simulink model "robot"  (R2021a)
settings: Solver=FixedStepAuto  StartTime=0.0  StopTime=tf  FixedStep=ts  RelTol=ts
PreLoadFcn:
  | robot_data;
InitFcn:
  | robot_data;
values from neighbouring files (symbols this model uses):
  c11 = coefficients_hexic(Theta(1,1), Theta(2,1), Theta(3,1), t1, tf)    [robot_data.m]
  c12 = NaN(size(c11))    [robot_data.m]
  c21 = coefficients_hexic(Theta(1,2), Theta(2,2), Theta(3,2), t1, tf)    [robot_data.m]
  c22 = NaN(size(c21))    [robot_data.m]
  obs = [0.2, 0.1]    [robot_data.m]
  offset = 0.183    [robot_data.m]
  r1 = 0.21    [robot_data.m]
  r2 = 0.2452    [robot_data.m]
  t1 = 4    [robot_data.m]    (also in trajectory_planning.m = 2)
settings Model: EnablePacing=on  Creator=matti  LastModifiedBy=matti

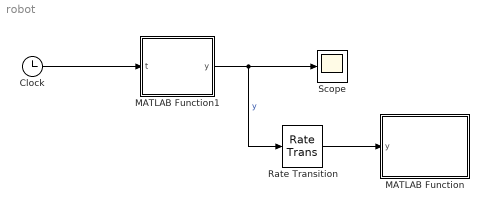
== system robot ==
  Clock : Clock
  MATLAB Function : MATLAB Function  TreatAsAtomicUnit=on
  MATLAB Function1 : MATLAB Function  TreatAsAtomicUnit=on
  Rate Transition : RateTransition  OutPortSampleTime=ts
  Scope : Scope
  wires:
  Rate Transition/1 -> MATLAB Function/1(y)
  Clock/1 -> MATLAB Function1/1(t)
  MATLAB Function1/1(y) -> Rate Transition/1, Scope/1  "y"

== matlab function robot/MATLAB Function ==
  data: y input; r1 parameter; r2 parameter; obs parameter; offset parameter
%% Animation function
function robot_display(y, r1, r2, obs, offset)
% Animation of the robot with the lower and upper arm as well as 
% the shoulder, elbow and hand and the obstacle
% Input     Type        Description
% y         2x1 double  simulation output
% Parameter Type        Description
% r1        1x1 double  upper arm length [m]
% r2        1x1 double  lower arm length [m]
% obs       2x1 double  x-position and height of the obstacle
% offset    1x1 double  y offset of first joint
coder.extrinsic('patch');
persistent upperarm;
persistent lowerarm;
persistent foot;
persistent shoulder;
persistent elbow;
persistent hand;
persistent obstacle;
%% Parameters
width = 0.02;      % width of both arms [m]
w2 = width/2;      % half of the width [m]
radius = 0.02;     % radius of joints [m]
%% Precalculation
s1 = sin(y(1));     % sine of theta1
c1 = cos(y(1));     % cosine of theta1
s12 = sin(y(1)+y(2));   % sine of theta1+theta2
c12 = cos(y(1)+y(2));   % cosine of theta1+theta2
xcu = -w2*s1;       % corner displacement upper arm in x
ycu = w2*c1;        % corner displacement upper arm in y
xcl = -w2*s12;      % corner displacement lower arm in x
ycl = w2*c12;       % corner displacement lower arm in y
x1 = c1*r1;         % elbow position in x
y1 = s1*r1;         % elbow position in y
x2 = x1+c12*r2;     % hand position in x
y2 = y1+s12*r2;     % hand position in y
%% Rectangle definition of foot, upper and lower arm
footx = [-width, -w2, w2, width];
footy = [0, offset, offset, 0];
upperarmx = [-xcu; xcu; x1+xcu; x1-xcu];
upperarmy = [-ycu; ycu; y1+ycu; y1-ycu]+offset;
lowerarmx = [x1-xcl; x1+xcl; x2+xcl; x2-xcl];
lowerarmy = [y1-ycl; y1+ycl; y2+ycl; y2-ycl]+offset;
%% Circle (octagon) definition of shoulder, elbow and hand
% modify for polygon with more corners
% alpha = 0:pi/4:7/4*pi;
% a = transpose(alpha);
% shoulderx = cos(a).*radius;
% shouldery = sin(a).*radius;
% octagon
r45 = radius/sqrt(2);   % value of x, y at 45° [m]
shoulderx = [radius; r45; 0; -r45; -radius; -r45; 0; r45];
shouldery = [0; r45; radius; r45; 0; -r45; -radius; -r45]+offset;
elbowx = shoulderx+x1;
elbowy = shouldery+y1;
handx = shoulderx+x2;
handy = shouldery+y2;
%% Obstacle definition
obstaclex = [obs(1)-w2, obs(1)-w2, obs(1)+w2, obs(1)+w2];
obstacley = [0, obs(2), obs(2), 0];
%% Animation
if isempty(lowerarm)% && isempty(upperarm) && isempty(shoulder) && isempty(elbow) && isempty(hand)
    figure(2);
    clf;
    title('Animation of the two-jointed robot');
    axis([-0.4 0.6 -0.2 0.8]);
    axis manual;
    grid on;
    hold on;
    upperarm = patch(upperarmx, upperarmy, zeros(4,1),...
        'FaceColor', 'b', 'EdgeColor', 'b');
    lowerarm = patch(lowerarmx, lowerarmy, zeros(4,1),...
        'FaceColor', 'b', 'EdgeColor', 'b');
    foot = patch(footx, footy, zeros(4,1),...
        'FaceColor', 'b', 'EdgeColor', 'b');
    shoulder = patch(shoulderx, shouldery, zeros(8,1),...
        'FaceColor', 'k', 'EdgeColor', 'k');
    elbow = patch(elbowx, elbowy, zeros(8,1),...
        'FaceColor', 'k', 'EdgeColor', 'k');
    hand = patch(handx, handy, zeros(8,1),...
        'FaceColor', 'k', 'EdgeColor', 'k');
    obstacle = patch(obstaclex, obstacley, zeros(4,1),...
        'FaceColor', 'r', 'EdgeColor', 'r');

end

set(upperarm, 'XData', upperarmx);
set(upperarm, 'YData', upperarmy);

set(lowerarm, 'XData', lowerarmx);
set(lowerarm, 'YData', lowerarmy);

% set(foot, 'XData', footx);
% set(foot, 'YData', footy);

% set(shoulder, 'XData', shoulderx);
% set(shoulder, 'YData', shouldery);

set(elbow, 'XData', elbowx);
set(elbow, 'YData', elbowy);

set(hand, 'XData', handx);
set(hand, 'YData', handy);

% set(obstacle, 'XData', obstaclex);
% set(obstacle, 'YData', obstacley);

end

== matlab function robot/MATLAB Function1 ==
  data: t input; y output; t1 parameter; c11 parameter; c21 parameter; c12 parameter; c22 parameter
%% Control function
function y = fcn(t,t1,c11,c21,c12,c22)
% Calculates the angles for each time step
% Input     Type        Description
% t         1x1 double  simulation time
% Parameter Type        Description
% c11       nx1 double  coefficients for joint 1 (to via)
% c21       nx1 double  coefficients for joint 2 (to via)
% c12       nx1 double  coefficients for joint 1 (from via)
% c22       nx1 double  coefficients for joint 2 (from via)
% t1        1x1 double  via time
% Output    Type        Description
% y         2x1 double  simulation output theta1 and theta2 [rad]

% Predefine output
y = zeros(2);
% Calculate trajectory for theta1 and theta2
if isnan(c12)
  y(1) = polyval(c11, t);
  y(2) = polyval(c21, t);
else
  if t <= t1
    y(1) = polyval(c11, t);
    y(2) = polyval(c21, t);
  else
    y(1) = polyval(c12, t-t1);
    y(2) = polyval(c22, t-t1);
  end
end
end
